simulink model "Example_2_Discretization_Mdl"  (Simulink 7.1)
settings: Solver=ode23s  StartTime=0.0  StopTime=5  RelTol=1e-3
values from neighbouring files (symbols this model uses):
  A = sys.a    [Example_2_Control.m]    (also in Example_2_Discretization.m; Example_2_Disturbance_Estimation.m; Example_2_Integral_Control.m; Example_2_Prediction_Observer.m)
  A_c = [0 1 0 -1; -k_s/m_s -b_s/m_s 0 b_s/m_s; 0 0 0 1; k_s/m_u b_s/m_u -k_u/m_u -b_s/m_u]    [Example_2_Analysis.m]    (also in Example_2_Control.m; Example_2_Discretization.m; Example_2_Disturbance_Estimation.m; Example_2_Integral_Control.m)
  a_ramp = 0.05    [Example_2_Control.m]    (also in Example_2_Discretization.m; Example_2_Integral_Control.m; Example_2_Prediction_Observer.m; Example_2_Reduced_Order_Observer.m)
  a_sin = 0.1    [Example_2_Control.m]    (also in Example_2_Discretization.m; Example_2_Integral_Control.m; Example_2_Prediction_Observer.m; Example_2_Reduced_Order_Observer.m)
  B = sys.b    [Example_2_Control.m]    (also in Example_2_Discretization.m; Example_2_Disturbance_Estimation.m; Example_2_Integral_Control.m; Example_2_Prediction_Observer.m)
  B_c = [0; 1/m_s; 0; -1/m_u]    [Example_2_Analysis.m]    (also in Example_2_Control.m; Example_2_Discretization.m; Example_2_Disturbance_Estimation.m; Example_2_Integral_Control.m)
  B_w = sys_d.b    [Example_2_Control.m]    (also in Example_2_Discretization.m; Example_2_Disturbance_Estimation.m; Example_2_Integral_Control.m; Example_2_Prediction_Observer.m)
  B_wc = [0; 0; -1; 0]    [Example_2_Analysis.m]    (also in Example_2_Control.m; Example_2_Discretization.m; Example_2_Disturbance_Estimation.m; Example_2_Integral_Control.m)
  C = sys.c    [Example_2_Control.m]    (also in Example_2_Discretization.m; Example_2_Disturbance_Estimation.m; Example_2_Integral_Control.m; Example_2_Prediction_Observer.m)
  C_c = [-k_s/m_s -b_s/m_s 0 b_s/m_s; 0 0 1 0]    [Example_2_Analysis.m]    (also in Example_2_Control.m; Example_2_Discretization.m; Example_2_Disturbance_Estimation.m = [-k_s/m_s -b_s/m_s 0 b_s/m_s]; Example_2_Integral_Control.m = [1 0 0 0])
  D = sys.d    [Example_2_Control.m]    (also in Example_2_Discretization.m; Example_2_Disturbance_Estimation.m; Example_2_Integral_Control.m; Example_2_Prediction_Observer.m)
  D_c = [1/m_s; 0]    [Example_2_Analysis.m]    (also in Example_2_Control.m; Example_2_Discretization.m; Example_2_Disturbance_Estimation.m = 0.0031746031746; Example_2_Integral_Control.m = 0)
  h = T_r/N_r    [Example_2_Control.m]    (also in Example_2_Discretization.m; Example_2_Disturbance_Estimation.m; Example_2_Integral_Control.m; Example_2_Prediction_Observer.m)
  l_ramp = 0.05    [Example_2_Control.m]    (also in Example_2_Discretization.m; Example_2_Integral_Control.m; Example_2_Prediction_Observer.m; Example_2_Reduced_Order_Observer.m)
  l_sin = 5    [Example_2_Control.m]    (also in Example_2_Discretization.m; Example_2_Integral_Control.m; Example_2_Prediction_Observer.m; Example_2_Reduced_Order_Observer.m)
  v = 40/3.6    (= 11.1111111111)    [Example_2_Control.m]    (also in Example_2_Discretization.m; Example_2_Disturbance_Estimation.m; Example_2_Integral_Control.m; Example_2_Prediction_Observer.m)
  x_0 = [0; 0; 0; 0]    [Example_2_Analysis.m]    (also in Example_2_Control.m = [25*9.81/k_s; 0; 25*9.81/k_u; 0]; Example_2_Discretization.m = [25*9.81/k_s; 0; 25*9.81/k_u; 0]; Example_2_Disturbance_Estimation.m; Example_2_Integral_Control.m)
libraries: simulink x1
settings Model: Creator=d_goerges  LastModifiedBy=d_goerges
settings DataIOCC: Refine=10
settings OptimizationCC: InitFltsAndDblsToZero=off
settings DebuggingCC: FcnCallInpInsideContextMsg=Enable All  StrictBusMsg=ErrorLevel1
settings GRTTargetCC: CPPClassGenCompliant=off

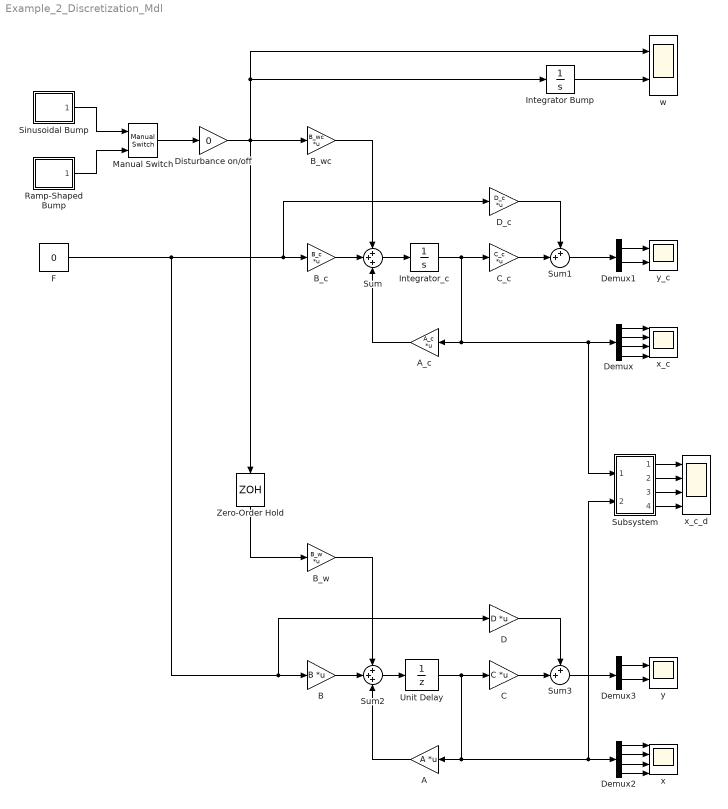
== system Example_2_Discretization_Mdl ==
  A : Gain  Orientation=left  Gain=A  Multiplication=Matrix(K*u)
  A_c : Gain  Orientation=left  Gain=A_c  Multiplication=Matrix(K*u)
  B : Gain  Gain=B  Multiplication=Matrix(K*u)
  B_c : Gain  Gain=B_c  Multiplication=Matrix(K*u)
  B_w : Gain  Gain=B_w  Multiplication=Matrix(K*u)  SampleTime=h
  B_wc : Gain  Gain=B_wc  Multiplication=Matrix(K*u)
  C : Gain  Gain=C  Multiplication=Matrix(K*u)
  C_c : Gain  Gain=C_c  Multiplication=Matrix(K*u)
  D : Gain  Gain=D  Multiplication=Matrix(K*u)
  D_c : Gain  Gain=D_c  Multiplication=Matrix(K*u)
  Demux : Demux
  Demux1 : Demux  Outputs=2
  Demux2 : Demux
  Demux3 : Demux  Outputs=2
  Disturbance on/off : Gain  Gain=0
  F : Constant  Value=0
  Integrator Bump : Integrator
  Integrator_c : Integrator  InitialCondition=x_0
  Manual Switch : simulink/Signal Routing/Manual Switch  sw=1  action=0  varsize=off
  Ramp-Shaped Bump : Subsystem
  Sinusoidal Bump : Subsystem
  Subsystem : Subsystem
  Sum : Sum  Inputs=+++
  Sum1 : Sum  Inputs=++|
  Sum2 : Sum  Inputs=+++
  Sum3 : Sum  Inputs=++|
  Unit Delay : UnitDelay  X0=x_0  SampleTime=h
  Zero-Order Hold : ZeroOrderHold  Orientation=down  SampleTime=h
  w : Scope  NumInputPorts=2
      settings: YMin=-5~-5  YMax=5~5  SaveName=ScopeData2
  x : Scope  NumInputPorts=4
      settings: YMin=-5~-5~-5~-5  YMax=5~5~5~5  SaveName=ScopeData5
  x_c : Scope  NumInputPorts=4
      settings: YMin=-5~-5~-5~-5  YMax=5~5~5~5
  x_c_d : Scope  NumInputPorts=4
      settings: TimeRange=5  YMin=-0.03~-0.4~-0.004~-0.2  YMax=0.05~0.3~0.01~0.5  SaveName=ScopeData3
  y : Scope  NumInputPorts=2
      settings: YMin=-5~-5  YMax=5~5  SaveName=ScopeData6
  y_c : Scope  NumInputPorts=2
      settings: YMin=-5~-5  YMax=5~5
  wires:
  Integrator_c/1 -> C_c/1, A_c/1, Demux/1, Subsystem/1(In1)
  Sum/1 -> Integrator_c/1
  F/1 -> B/1, D/1, B_c/1, D_c/1
  B_c/1 -> Sum/2
  A_c/1 -> Sum/3
  B_wc/1 -> Sum/1
  C_c/1 -> Sum1/2
  D_c/1 -> Sum1/1
  Demux/1 -> x_c/1
  Demux/2 -> x_c/2
  Demux/3 -> x_c/3
  Demux/4 -> x_c/4
  Sum1/1 -> Demux1/1
  Demux1/1 -> y_c/1
  Demux1/2 -> y_c/2
  Sum2/1 -> Unit Delay/1
  B/1 -> Sum2/2
  A/1 -> Sum2/3
  B_w/1 -> Sum2/1
  C/1 -> Sum3/2
  D/1 -> Sum3/1
  Demux2/1 -> x/1
  Demux2/2 -> x/2
  Demux2/3 -> x/3
  Demux2/4 -> x/4
  Sum3/1 -> Demux3/1
  Demux3/1 -> y/1
  Demux3/2 -> y/2
  Subsystem/1(Out1) -> x_c_d/1
  Subsystem/2(Out2) -> x_c_d/2
  Subsystem/3(Out3) -> x_c_d/3
  Subsystem/4(Out4) -> x_c_d/4
  Manual Switch/1 -> Disturbance on/off/1
  Unit Delay/1 -> A/1, Demux2/1, Subsystem/2(In2), C/1
  Sinusoidal Bump/1(z_r_dot) -> Manual Switch/1
  Ramp-Shaped Bump/1(z_r_dot) -> Manual Switch/2
  Integrator Bump/1 -> w/2
  Zero-Order Hold/1 -> B_w/1
  Disturbance on/off/1 -> B_wc/1, w/1, Integrator Bump/1, Zero-Order Hold/1

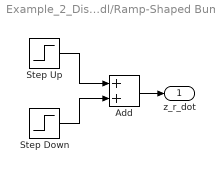
== system Example_2_Discretization_Mdl/Ramp-Shaped Bump ==
  Add : Sum
  Step Down : Step  Time=l_ramp/v  After=-a_ramp/l_ramp*v  SampleTime=0
  Step Up : Step  Time=0  After=a_ramp/l_ramp*v  SampleTime=0
  z_r_dot : Outport
  wires:
  Step Up/1 -> Add/1
  Step Down/1 -> Add/2
  Add/1 -> z_r_dot/1

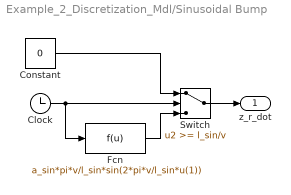
== system Example_2_Discretization_Mdl/Sinusoidal Bump ==
  Clock : Clock
  Constant : Constant  Value=0
  Fcn : Fcn  Expr=a_sin*pi*v/l_sin*sin(2*pi*v/l_sin*u(1))
  Switch : Switch  Threshold=l_sin/v
  z_r_dot : Outport
  wires:
  Switch/1 -> z_r_dot/1
  Fcn/1 -> Switch/3
  Constant/1 -> Switch/1
  Clock/1 -> Fcn/1, Switch/2

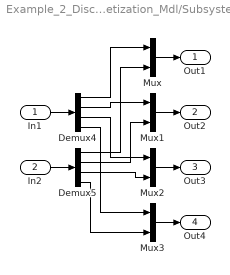
== system Example_2_Discretization_Mdl/Subsystem ==
  In1 : Inport
  In2 : Inport  Port=2
  Demux4 : Demux
  Demux5 : Demux
  Mux{,1..3} (4 alike) : Mux  Inputs=2
  Out1 : Outport
  Out2 : Outport  Port=2
  Out3 : Outport  Port=3
  Out4 : Outport  Port=4
  wires:
  Demux4/1 -> Mux/1
  Demux4/2 -> Mux1/1
  Demux4/3 -> Mux2/1
  Demux4/4 -> Mux3/1
  Demux5/1 -> Mux/2
  Demux5/2 -> Mux1/2
  Demux5/3 -> Mux2/2
  Demux5/4 -> Mux3/2
  Mux/1 -> Out1/1
  In1/1 -> Demux4/1
  Mux1/1 -> Out2/1
  In2/1 -> Demux5/1
  Mux2/1 -> Out3/1
  Mux3/1 -> Out4/1
